simulink model "sl_braitenberg"  (R2023a)
settings: Solver=VariableStepAuto  StartTime=0.0  StopTime=200  RelTol=1e-3
undefined symbols (not defined in the file or in its folder): rotm2d, se2
libraries: robotmobilelib x1
Description:
  | Drive a vehicle toward the maximum of a scalar field.
  | 
  | Robotics, Vision and Control - 3rd Edition; Section 5.1.1
settings Model: Creator=rpill  LastModifiedBy=rpillat
settings SolverCC: AlgebraicLoopSolver=TrustRegion  MaxZcPerStep=1
settings DataIOCC: DSMLogging=off  TimeSaveName=t  OutputSaveName=y
settings OptimizationCC: ReuseModelBlockBuffer=off
settings DebuggingCC: UnconnectedInputMsg=warning  UnconnectedOutputMsg=warning  UnconnectedLineMsg=warning
settings ModelReferenceCC: EnableRefExpFcnMdlSchedulingChecks=on
settings RTWCC: DLArmComputeVersion=19.05

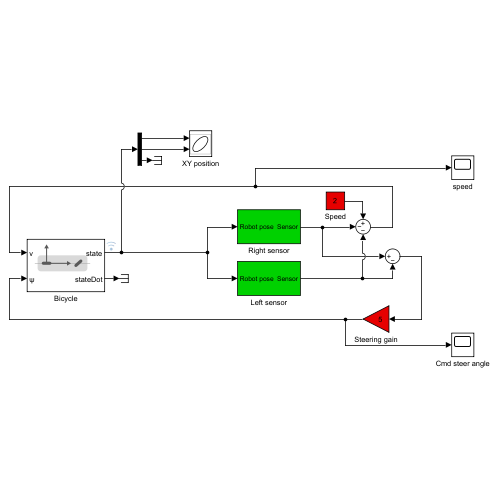
[thumbnail: Simulink's stored preview of the top-level diagram]
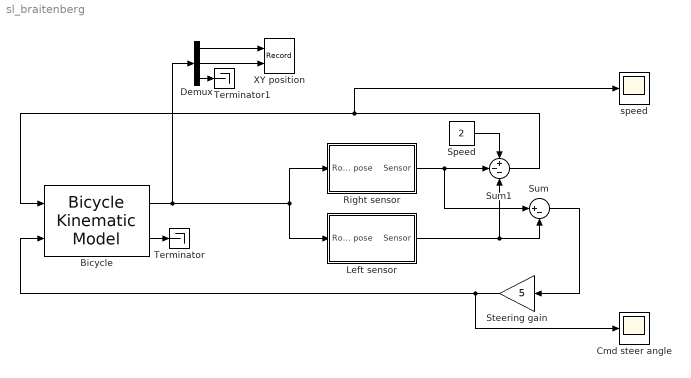
== system sl_braitenberg ==
  Bicycle : robotmobilelib/Bicycle Kinematic Model  VehicleInputs=Vehicle Speed & Steering Angle  WheelBase=1  VehicleSpeedRange=[-1 1]  MaxSteeringAngle=pi/4  InitialState=[0; 0; 0]  SimulateUsing=Interpreted execution
  Cmd steer angle : Scope
  Demux : Demux  Outputs=3
  Left sensor : Subsystem  mask{dx=0, dy=-2, sensorfunc=@sensorfield}
      mask prompts: dx "Sensor position x"; dy "Sensor position y"; sensorfunc "Sensor function"
  Right sensor : Subsystem  mask{dx=0, dy=2, sensorfunc=@sensorfield}
      mask prompts: dx "Sensor position x"; dy "Sensor position y"; sensorfunc "Sensor function"
  Speed : Constant  Value=2
  Steering gain : Gain  Gain=5
  Sum : Sum  Inputs=|+-
  Sum1 : Sum  Inputs=+--
  Terminator : Terminator
  Terminator1 : Terminator
  XY position : Record  FileSettingsInternal="{\"entries\":[{\"content\":{\"excelSettings\":{\"content\":{},\"type\":\"Streamout.ExcelSettings\"}},\"type\":\"Streamout.FileSettingStorage\",\"uuid\":\"81c345f8-3c27-48e9-874c-ad1f089ddf81\"}],\"packageUris\":[\"http://schema.mathworks.com/mf0/streamout_blocks/R2020a\"],\"version\":\"1.0\"}"  Layout=[1 1]  SignalsInternal="{\"entries\":[{\"content\":{\"signals\":[{\"content\":{\"blockPath\":[\"sl_braitenberg/XY position\"],\"channel\":[],\"dimensions\":[1],\"domain\":\"sl_braitenberg/XY position\",\"lineColor\":\"#a2142f\",\"plots\":[1],\"port\":1,\"sid\":[],\"signalID\":8,\"signalName\":\"Demux:1\"},\"type\":\"RecordBlkView.Signal\",\"uuid\":\"873fdd24-6a9f-401a-b933-91c7ab0dee13\"},{\"content\":{\"blockPath\":[\"sl_braitenberg/XY position\"],\"channel\":[],\"dimensions\":[1],\"domain\":\"sl_braitenberg/XY position\",\"lineColor\":\"#139fff\",\"plots\":[1],\"port\":2,\"sid\":[],\"signalID\":11,\"signalName\":\"Demux:2\"},\"type\":\"RecordBlkView.Signal\",\"uuid\":\"883bfaec-f233-4c84-96d1-b2d0e4fa6281\"}]},\"type\":\"RecordBlkView.InputSignals\",\"uuid\":\"6b83e4f7-b4e2-4ddf-a4bb-b2f340755928\"}],\"packageUris\":[\"http://schema.mathworks.com/mf0/streamout_blocks/R2020a\"],\"version\":\"1.0\"}"  VisualizationBindings="{\"xyplotplugin\":{\"info\":[{\"series\":[{\"bindingParametersList\":[{\"parameter\":\"X-Axis\",\"signalID\":8,\"signalName\":\"Demux:1\"},{\"parameter\":\"Y-Axis\",\"signalID\":11,\"signalName\":\"Demux:2\"}],\"seriesID\":1325}],\"subplotID\":1}]}}"  CompatibilityTag=XY  st=-1
  speed : Scope
  wires:
  Sum/1 -> Steering gain/1
  Speed/1 -> Sum1/1
  Left sensor/1(Sensor) -> Sum/2, Sum1/3
  Steering gain/1 -> Cmd steer angle/1, Bicycle/2
  Sum1/1 -> Bicycle/1, speed/1
  Bicycle/1 -> Demux/1, Right sensor/1(Robot pose), Left sensor/1(Robot pose)
  Right sensor/1(Sensor) -> Sum/1, Sum1/2
  Bicycle/2 -> Terminator/1
  Demux/1 -> XY position/1
  Demux/2 -> XY position/2
  Demux/3 -> Terminator1/1

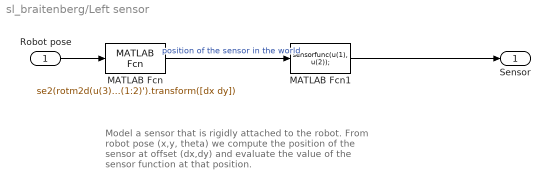
== system sl_braitenberg/Left sensor ==
  note: Model a sensor that is rigidly attached to the robot.
      | From robot pose (x,y, theta) we compute the position of
      | the sensor at offset (dx,dy) and evaluate the value
      | of the sensor function at that position.
  Robot pose : Inport
  MATLAB Fcn : MATLABFcn  MATLABFcn=se2(rotm2d(u(3)),u(1:2)').transform([dx dy])
  MATLAB Fcn1 : MATLABFcn  MATLABFcn=sensorfunc(u(1), u(2));  OutputDimensions=1
  Sensor : Outport
  wires:
  Robot pose/1 -> MATLAB Fcn/1
  MATLAB Fcn/1 -> MATLAB Fcn1/1  "position of the sensor in the world"
  MATLAB Fcn1/1 -> Sensor/1

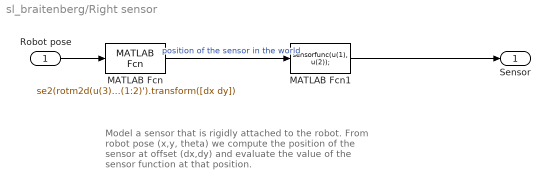
== system sl_braitenberg/Right sensor ==
  note: Model a sensor that is rigidly attached to the robot.
      | From robot pose (x,y, theta) we compute the position of
      | the sensor at offset (dx,dy) and evaluate the value
      | of the sensor function at that position.
  Robot pose : Inport
  MATLAB Fcn : MATLABFcn  MATLABFcn=se2(rotm2d(u(3)),u(1:2)').transform([dx dy])
  MATLAB Fcn1 : MATLABFcn  MATLABFcn=sensorfunc(u(1), u(2));  OutputDimensions=1
  Sensor : Outport
  wires:
  Robot pose/1 -> MATLAB Fcn/1
  MATLAB Fcn/1 -> MATLAB Fcn1/1  "position of the sensor in the world"
  MATLAB Fcn1/1 -> Sensor/1
